simulink model "psk_2"  (Simulink 5.1)
settings: Solver=ode45  StartTime=0.0  StopTime=2  RelTol=1e-3
values from neighbouring files (symbols this model uses):
  fc = 0.2    [TP_fdesign1.m]    (also in TP_fdesign2.m; band4.m = 2000)
  M = 2    [CFIR_1.m]    (also in block_lms_.m = 16; cic_dezim1.m = ',num2str(M),'; cic_dezim1_.m = ',num2str(M),     '; cic_dezim2.m = ',num2str(M),')
  nf = 256    [band4.m]    (also in block_lms_.m = 16)
  Ts = 1/fs    (= 6.25e-05)    [G722_1.m]    (also in adaptiv_2.m = 0.001; adaptiv_3.m = 0.001; adaptiv_4.m = 0.001; adaptiv_5.m = 0.001)
undefined symbols (not defined in the file or in its folder): get, gt
libraries: dspbuff3 x2, dspsigops x2, dspsigattribs x2, dspmtrx3 x2, dspsrcs4 x1, dspsnks4 x1
settings Model: Creator=svenhoffmann  LastModifiedBy=svenhoffmann  ExtModeAutoUpdateStatusClock=off  BooleanDataType=on  ProdHWDeviceType=Microprocessor

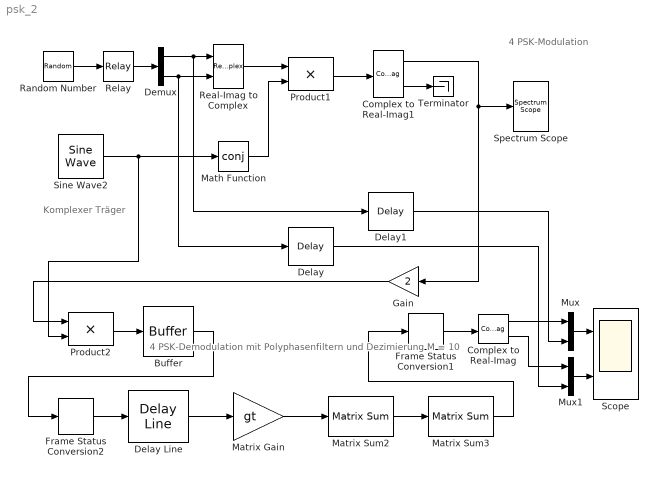
== system psk_2 ==
  note: 4 PSK-Modulation
  note: Komplexer
      | Träger
  note: 4 PSK-Demodulation
      | mit Polyphasenfiltern
      | und Dezimierung
      | M = 10
  Buffer : dspbuff3/Buffer  N=M  V=0  ic=0
  Complex to Real-Imag : ComplexToRealImag
  Complex to Real-Imag1 : ComplexToRealImag
  Delay : dspsigops/Delay  dly_unit=Samples  delay=nf/2  ic_detail=off  dif_ic_for_ch=off  dif_ic_for_dly=off  ic=0  reset_popup=None
  Delay Line : dspbuff3/Delay Line  siz=ng  ic=0  directfeed=off
  Delay1 : dspsigops/Delay  dly_unit=Samples  delay=nf/2  ic_detail=off  dif_ic_for_ch=off  dif_ic_for_dly=off  ic=0  reset_popup=None
  Demux : Demux  Outputs=2
  Frame Status Conversion1 : dspsigattribs/Frame Status Conversion  growRefPort=off  outframe=Sample-based
  Frame Status Conversion2 : dspsigattribs/Frame Status Conversion  growRefPort=off  outframe=Sample-based
  Gain : Gain  Orientation=left  Gain=2  SaturateOnIntegerOverflow=on
  Math Function : Math  Operator=conj
  Matrix Gain : Gain  Gain=gt  SaturateOnIntegerOverflow=on
  Matrix Sum2 : dspmtrx3/Matrix Sum  Dim=Columns  roundingMode=Floor  overflowMode=off
  Matrix Sum3 : dspmtrx3/Matrix Sum  Dim=Rows  roundingMode=Floor  overflowMode=off
  Mux : Mux  Inputs=2
  Mux1 : Mux  Inputs=2
  Product1 : Product  SaturateOnIntegerOverflow=on
  Product2 : Product  SaturateOnIntegerOverflow=on
  Random Number : RandomNumber  Seed=[0124, 769]  SampleTime=100*Ts
  Real-Imag to Complex : RealImagToComplex
  Relay : Relay  OffOutputValue=-1  SampleTime=Ts
  Scope : Scope  NumInputPorts=2
      settings: YMin=-1~-1  YMax=1~1
  Sine Wave2 : dspsrcs4/Sine Wave  Amplitude=1  Frequency=fc  Phase=0  SampleMode=Discrete  OutComplex=Complex  CompMethod=Trigonometric fcn  TableSize=Speed  SampleTime=Ts  SamplesPerFrame=1  dataType=double  wordLen=16  udDataType=sfix(16)  fracBitsMode=Best precision  numFracBits=15  ResetState=Restart at time zero
      settings: additionalParams=on
  Spectrum Scope : dspsnks4/Spectrum Scope  ScopeProperties=off  Domain=Frequency  HorizSpan=1  UseBuffer=on  BufferSize=256  Overlap=64  inpFftLenInherit=off  FFTlength=128  numAvg=10  DisplayProperties=off  AxisGrid=on  Memory=off  FrameNumber=on  AxisLegend=off  AxisZoom=off  OpenScopeAtSimStart=on  OpenScopeImmediately=off  FigPos=get(0,'defaultfigureposition')  AxisProperties=on  XUnits=Hertz  XRange=[0...Fs]  InheritXIncr=off  XIncr=Ts  XLabel=Samples  YUnits=dB  YLabel=Magnitude, dB  LineProperties=off
      settings: YMin=-27.4679460175424  YMax=16.0428342016301
  Terminator : Terminator
  wires:
  Mux/1 -> Scope/1
  Random Number/1 -> Relay/1
  Sine Wave2/1 -> Product2/2, Math Function/1
  Product1/1 -> Complex to Real-Imag1/1
  Complex to Real-Imag1/1 -> Spectrum Scope/1, Gain/1
  Complex to Real-Imag1/2 -> Terminator/1
  Relay/1 -> Demux/1
  Demux/1 -> Real-Imag to Complex/1, Delay1/1
  Demux/2 -> Real-Imag to Complex/2, Delay/1
  Real-Imag to Complex/1 -> Product1/1
  Mux1/1 -> Scope/2
  Delay/1 -> Mux1/2
  Delay1/1 -> Mux/2
  Complex to Real-Imag/1 -> Mux/1
  Complex to Real-Imag/2 -> Mux1/1
  Buffer/1 -> Frame Status Conversion2/1
  Product2/1 -> Buffer/1
  Delay Line/1 -> Matrix Gain/1
  Matrix Sum2/1 -> Matrix Sum3/1
  Matrix Gain/1 -> Matrix Sum2/1
  Matrix Sum3/1 -> Frame Status Conversion1/1
  Frame Status Conversion1/1 -> Complex to Real-Imag/1
  Frame Status Conversion2/1 -> Delay Line/1
  Math Function/1 -> Product1/2
  Gain/1 -> Product2/1
